simulink model "lab01fig01"  (R2015a)
settings: Solver=ode45  StartTime=0.0  StopTime=10.0  RelTol=1e-3
settings Model: Creator=dg  LastModifiedBy=dg

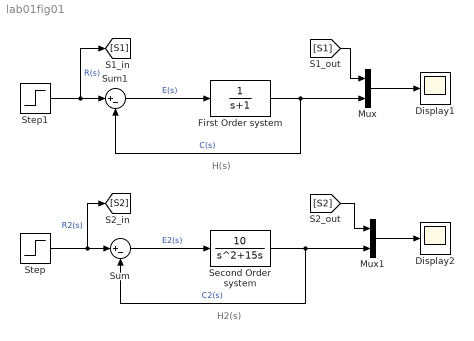
== system lab01fig01 ==
  note: H2(s)
  note: H(s)
  Display1 : Scope
      settings: TimeRange=10  YMin=0  YMax=1.15  ScrollMode=on
  Display2 : Scope
      settings: YMin=0  YMax=1.15
  First Order system : TransferFcn  Denominator=[1 1]
  Mux : Mux  Inputs=2
  Mux1 : Mux  Inputs=2
  Second Order system : TransferFcn  Numerator=[10]  Denominator=[1 15 0]
  Step : Step  Time=0  SampleTime=0
  Step1 : Step  Time=0  SampleTime=0
  Sum : Sum  Inputs=|+-
  Sum1 : Sum  Inputs=|+-
  wires:
  Step/1 -> [S2], Sum/1  "R2(s)"
  Sum/1 -> Second Order system/1  "E2(s)"
  Second Order system/1 -> Mux1/2, Sum/2  "C2(s)"
  Step1/1 -> [S1], Sum1/1  "R(s)"
  Sum1/1 -> First Order system/1  "E(s)"
  First Order system/1 -> Mux/2, Sum1/2  "C(s)"
  Mux/1 -> Display1/1
  Mux1/1 -> Display2/1
  [S1] -> Mux/1
  [S2] -> Mux1/1
